simulink model "FSK_2024b"  (R2024b)
settings: Solver=VariableStepDiscrete  StartTime=0.0  StopTime=2000/Rb  RelTol=1e-3  EnableMultiTasking=on
PreLoadFcn:
  | fc=30000;
  | Rb=9600;
  | df=Rb;
libraries: commrandsrc3 x1
settings Model: Creator=morelos_zaragoza  LastModifiedBy=14083
settings SolverCC: AlgebraicLoopSolver=TrustRegion
settings DataIOCC: LimitDataPoints=on  SaveFormat=Array  SignalLoggingSaveFormat=ModelDataLogs  ReturnWorkspaceOutputs=off
settings OptimizationCC: ExpressionDepthLimit=2147483647  InitFltsAndDblsToZero=on  LifeSpan=inf
settings DebuggingCC: SaveWithParameterizedLinksMsg=none  UnderspecifiedInitializationDetection=Classic  MergeDetectMultiDrivingBlocksExec=none  SignalResolutionControl=TryResolveAllWithWarning  SolverPrmCheckMsg=warning  MultiTaskDSMMsg=warning  MultiTaskCondExecSysMsg=none  FcnCallInpInsideContextMsg=warning  UnconnectedInputMsg=warning  UnconnectedOutputMsg=warning  UnconnectedLineMsg=warning  StateNameClashWarn=warning  SFUnexpectedBacktrackingDiag=warning  SFNoUnconditionalDefaultTransitionDiag=warning  SFExecutionAtInitializationDiag=none  ArithmeticOperatorsInVariantConditions=warning
settings HardwareCC: ProdBitPerPointer=32  ProdBitPerSizeT=32  ProdBitPerPtrDiffT=32  ProdLargestAtomicFloat=None  ProdIntDivRoundTo=Undefined  ProdEndianess=Unspecified  ProdWordSize=32  ProdHWDeviceType=32-bit Generic
settings ModelReferenceCC: EnableRefExpFcnMdlSchedulingChecks=on  PropagateSignalLabelsOutOfModel=off
settings SFSimCC: SimUseLocalCustomCode=off  CustomCodeUndefinedFunction=UseInterfaceOnly
settings RTWCC: RTWUseLocalCustomCode=off  GPUComputeCapability=3.5
settings CodeAppCC: StateflowObjectComments=on
settings GRTTargetCC: TargetFcnLib=ansi_tfl_tmw.mat  TargetLangStandard=C89/C90 (ANSI)  CombineOutputUpdateFcns=off  GRTInterface=on
settings ConfigComp: CovMetricSettings=dw  CovSaveCumulativeToWorkspaceVar=on  CovSaveSingleToWorkspaceVar=on  CovExternalEMLEnable=off

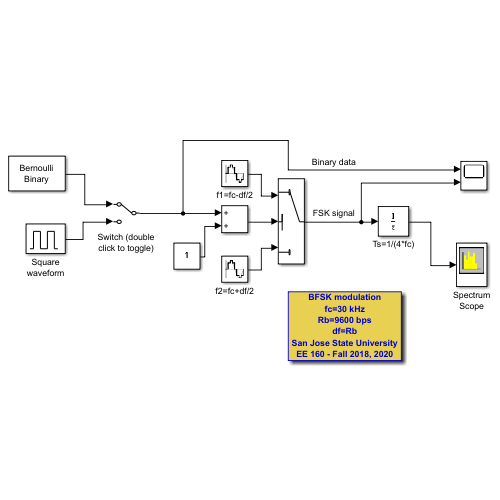
[thumbnail: Simulink's stored preview of the top-level diagram]
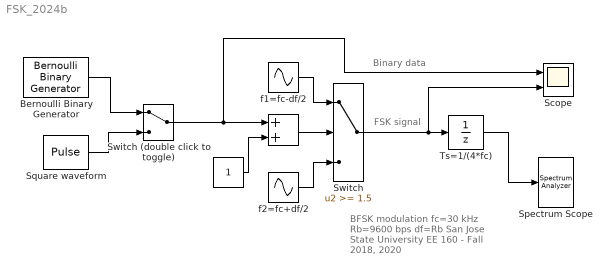
== system FSK_2024b ==
  note: FSK signal
  note: Binary data
  note: BFSK modulation
      | fc=30 kHz
      | Rb=9600 bps
      | df=Rb
      | San Jose State University
      | EE 160 - Fall 2018, 2020
  " " : Constant
  "  " : Sum
  Bernoulli Binary Generator : commrandsrc3/Bernoulli Binary Generator  ProbabilityOfZero=0.5  SeedSource=Auto  Seed=0  SampleTime=1/(4*Rb)  SamplesPerFrame=1  OutputDataType=double  SimulateUsing=Interpreted execution
  Scope : Scope  NumInputPorts=2
  Spectrum Scope : SpectrumAnalyzer  WindowPosition=[767.000000,69.000000,522.000000,333.000000,]  Visible=on  ScopeFrameLocation=window  Method=Welch  SampleRate=120000  PlotAsTwoSidedSpectrum=off  AxesScaling=Manual  FrequencyResolutionMethod=Window length  WindowLength=512  FFTLengthSource=Property  FFTLength=512  Span=60000  CenterFrequency=30000  StartFrequency=0  StopFrequency=60000  OverlapPercent=25  AveragingMethod=Running  SpectralAverages=100  YLabel=Magnitude  YLimits=[-15,25]  AllowFFTLengthLessThanSamplesPerUpdate=on  DefaultConfigurationName=spbscopes.SpectrumAnalyzerBlockCfg  IsFrequencyInputMode=0  FrequencyVectorPort=0  FrequencyVectorFromPort=0  FrequencyInputRBWPort=0  FrequencyInputRBWFromPort=0  SegLen=512
  Square waveform : DiscretePulseGenerator  PulseType=Time based  Period=2/Rb  PulseWidth=50
  Switch : Switch  Threshold=1.5  SaturateOnIntegerOverflow=off  InputSameDT=off
  Switch (double click to toggle) : ManualSwitch
  Ts=1/(4*fc) : UnitDelay  SampleTime=1/(4*fc)  HasFrameUpgradeWarning=on
  f1=fc-df/2 : Sin  Frequency=2*pi*(fc-df/2)  SampleTime=1/(16*fc)
  f2=fc+df/2 : Sin  Frequency=2*pi*(fc+df/2)  SampleTime=1/(16*fc)
  wires:
  f1=fc-df/2/1 -> Switch/1
  f2=fc+df/2/1 -> Switch/3
  " "/1 -> "  "/2
  "  "/1 -> Switch/2
  Switch/1 -> Ts=1/(4*fc)/1, Scope/2
  Ts=1/(4*fc)/1 -> Spectrum Scope/1
  Square waveform/1 -> Switch (double click to toggle)/2
  Bernoulli Binary Generator/1 -> Switch (double click to toggle)/1
  Switch (double click to toggle)/1 -> Scope/1, "  "/1
